simulink model "Recitifers"  (R2018a)
settings: Solver=VariableStepAuto  StartTime=0.0  StopTime=10  RelTol=1e-3
settings Model: Creator=Abhishek Srivastava  LastModifiedBy=Abhishek Srivastava

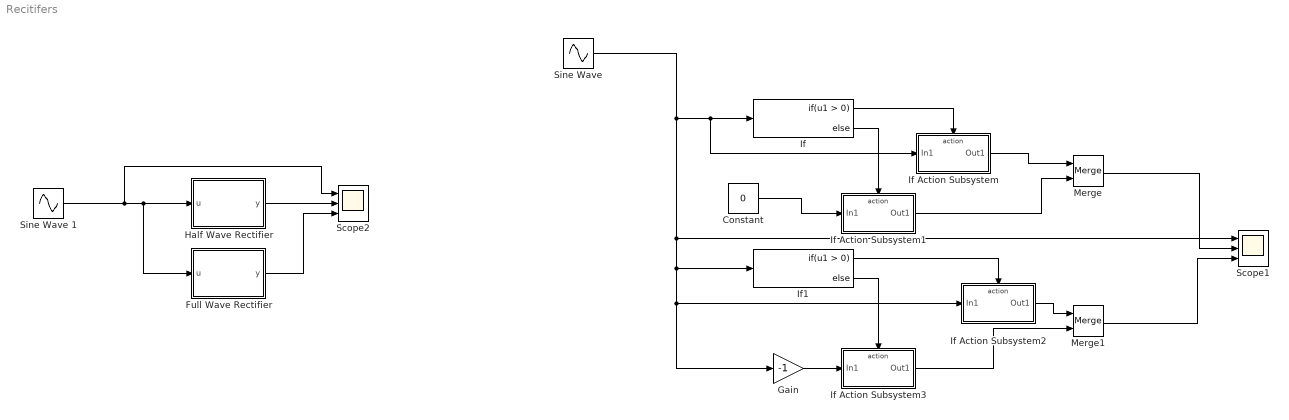
== system Recitifers ==
  Constant : Constant  Value=0
  Full Wave Rectifier : MATLAB Function  TreatAsAtomicUnit=on
  Gain : Gain  Gain=-1
  Half Wave Rectifier : MATLAB Function  TreatAsAtomicUnit=on
  If : If
  If Action Subsystem : Subsystem  TreatAsAtomicUnit=on
  If Action Subsystem1 : Subsystem  TreatAsAtomicUnit=on
  If Action Subsystem2 : Subsystem  TreatAsAtomicUnit=on
  If Action Subsystem3 : Subsystem  TreatAsAtomicUnit=on
  If1 : If
  Merge : Merge
  Merge1 : Merge
  Scope1 : Scope  NumInputPorts=3
  Scope2 : Scope  NumInputPorts=3
  "Sine Wave " : Sin  SampleTime=0
  Sine Wave 1 : Sin  SampleTime=0
  wires:
  "Sine Wave "/1 -> Scope1/1, If1/1, Gain/1, If Action Subsystem2/1(In1), If Action Subsystem/1(In1), If/1
  If/1 -> If Action Subsystem/Action
  If/2 -> If Action Subsystem1/Action
  If Action Subsystem/1(Out1) -> Merge/1
  If Action Subsystem1/1(Out1) -> Merge/2
  If Action Subsystem2/1(Out1) -> Merge1/1
  Merge/1 -> Scope1/2
  Merge1/1 -> Scope1/3
  If1/1 -> If Action Subsystem2/Action
  If1/2 -> If Action Subsystem3/Action
  Constant/1 -> If Action Subsystem1/1(In1)
  If Action Subsystem3/1(Out1) -> Merge1/2
  Gain/1 -> If Action Subsystem3/1(In1)
  Sine Wave 1/1 -> Scope2/1, Half Wave Rectifier/1(u), Full Wave Rectifier/1(u)
  Half Wave Rectifier/1(y) -> Scope2/2
  Full Wave Rectifier/1(y) -> Scope2/3

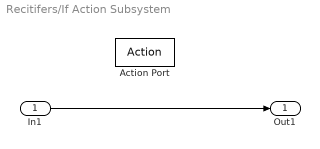
== system Recitifers/If Action Subsystem ==
  In1 : Inport
  Action Port : ActionPort  ActionType=then
  Out1 : Outport
  wires:
  In1/1 -> Out1/1

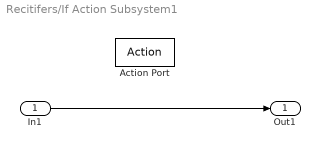
== system Recitifers/If Action Subsystem1 ==
  In1 : Inport
  Action Port : ActionPort  ActionType=else
  Out1 : Outport
  wires:
  In1/1 -> Out1/1

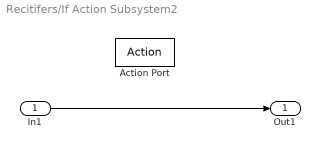
== system Recitifers/If Action Subsystem2 ==
  In1 : Inport
  Action Port : ActionPort  ActionType=then
  Out1 : Outport
  wires:
  In1/1 -> Out1/1

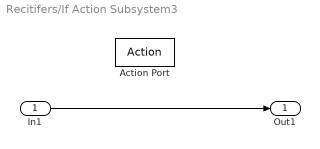
== system Recitifers/If Action Subsystem3 ==
  In1 : Inport
  Action Port : ActionPort  ActionType=else
  Out1 : Outport
  wires:
  In1/1 -> Out1/1

== matlab function Recitifers/Half Wave Rectifier ==
  data: u input; y output
function y = fcn(u)
    if u<0
        y=0;
   else
        y = u;   
   end

== matlab function Recitifers/Full Wave Rectifier ==
  data: u input; y output
function y = fcn(u)
    if u<0
        y=-u;
   else
        y = u;   
   end
